simulink model "BLDC_full_sysid"  (R2024b)
settings: Solver=ode4  StartTime=0.0  StopTime=10.0  FixedStep=0.0001  RelTol=1e-3
values from neighbouring files (symbols this model uses):
  d = 0.35757    [DRBA_motor_EKF.m]    (also in DRBA_motor_PID_control.m; DRBA_motor_sysid.m = 0.1)
  f = 0.53378    [DRBA_motor_EKF.m]    (also in DRBA_motor_PID_control.m; DRBA_motor_sysid.m = 0.05)
  J = 0.05    [DRBA_motor_EKF.m]    (also in DRBA_motor_PID_control.m; DRBA_motor_sysid.m = 0.03)
  Kb = 20.91    [DRBA_motor_EKF.m]    (also in DRBA_motor_PID_control.m; DRBA_motor_sysid.m = 22)
  Kt = 0.7    [DRBA_motor_EKF.m]    (also in DRBA_motor_PID_control.m; DRBA_motor_sysid.m = 0.72)
  L = 0.00069    [DRBA_motor_EKF.m]    (also in DRBA_motor_PID_control.m; DRBA_motor_sysid.m = 0.00067)
  R = 0.0755    [DRBA_motor_EKF.m]    (also in DRBA_motor_PID_control.m; DRBA_motor_sysid.m = 0.0725)
settings Model: Creator=User  LastModifiedBy=User

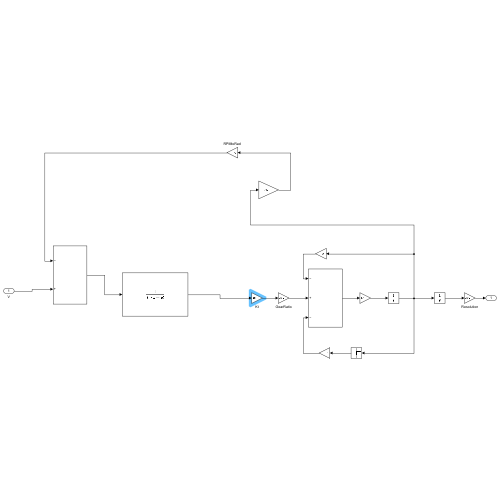
[thumbnail: Simulink's stored preview of the top-level diagram]
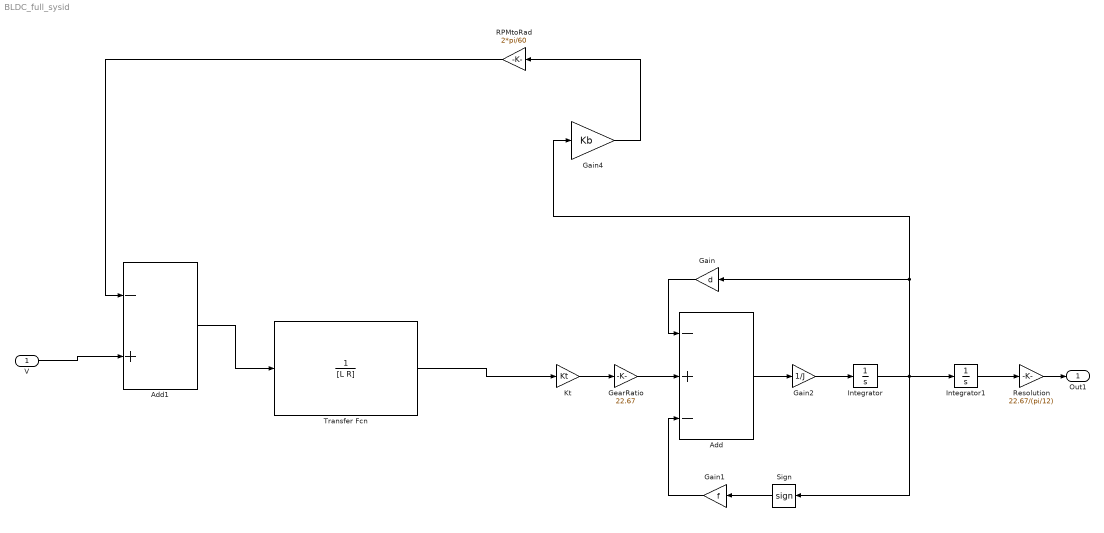
== system BLDC_full_sysid ==
  V : Inport
  Add : Sum  Inputs=-+-
  Add1 : Sum  Inputs=-+
  Gain : Gain  Gain=d
  Gain1 : Gain  Gain=f
  Gain2 : Gain  Gain=1/J
  Gain4 : Gain  Gain=Kb
  GearRatio : Gain  Gain=22.67
  Integrator : Integrator
  Integrator1 : Integrator
  Kt : Gain  Gain=Kt
  RPMtoRad : Gain  Gain=2*pi/60
  Resolution : Gain  Gain=22.67/(pi/12)  RndMeth=Zero  SaturateOnIntegerOverflow=on
  Sign : Signum  ZeroCross=off
  Transfer Fcn : TransferFcn  Denominator=[L R]
  Out1 : Outport
  wires:
  Resolution/1 -> Out1/1
  Integrator1/1 -> Resolution/1
  Gain/1 -> Add/1
  Add/1 -> Gain2/1
  Kt/1 -> GearRatio/1
  GearRatio/1 -> Add/2
  Gain2/1 -> Integrator/1
  Integrator/1 -> Integrator1/1, Gain4/1, Gain/1, Sign/1
  Gain1/1 -> Add/3
  Sign/1 -> Gain1/1
  Transfer Fcn/1 -> Kt/1
  V/1 -> Add1/2
  Add1/1 -> Transfer Fcn/1
  Gain4/1 -> RPMtoRad/1
  RPMtoRad/1 -> Add1/1
